simulink model "Fluid_Power_Control"  (R2024b)
settings: Solver=VariableStepAuto  StartTime=0.0  StopTime=10.0  RelTol=1e-3
model workspace (MAT data in the model file):
  b = 3
  m = 3
undefined symbols (not defined in the file): A, B, FL, kc, kq, ms, V
settings Model: Creator=audreyday  LastModifiedBy=audreyday

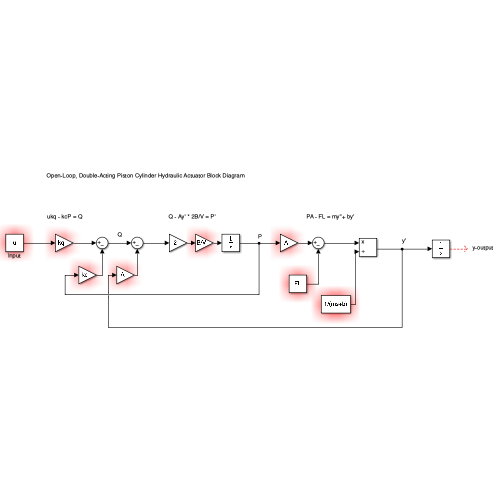
[thumbnail: Simulink's stored preview of the top-level diagram]
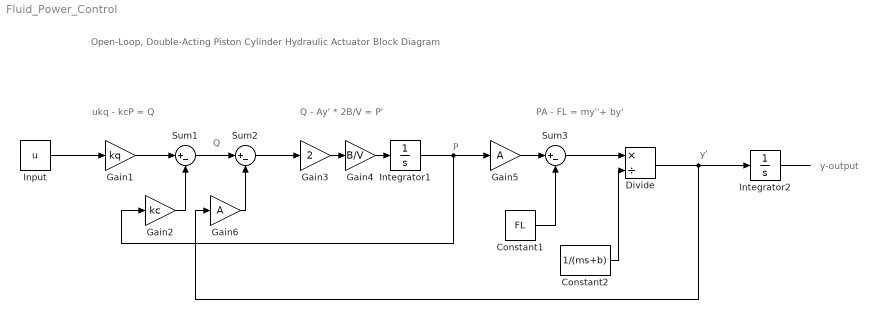
== system Fluid_Power_Control ==
  note: Open-Loop, Double-Acting Piston Cylinder Hydraulic Actuator Block Diagram
  note: y'
  note: PA - FL = my''+ by'
  note: P
  note: Q - Ay' * 2B/V = P'
  note: y-output
  note: ukq - kcP = Q
  note: Q
  Constant1 : Constant  Value=FL
  Constant2 : Constant  Value=1/(ms+b)
  Divide : Product  Inputs=*/
  Gain1 : Gain  Gain=kq
  Gain2 : Gain  Gain=kc
  Gain3 : Gain  Gain=2
  Gain4 : Gain  Gain=B/V
  Gain5 : Gain  Gain=A
  Gain6 : Gain  Gain=A
  Input : Constant  Value=u
  Integrator1 : Integrator
  Integrator2 : Integrator
  Sum1 : Sum  Inputs=|+-
  Sum2 : Sum  Inputs=|+-
  Sum3 : Sum  Inputs=|+-
  wires:
  Input/1 -> Gain1/1
  Gain1/1 -> Sum1/1
  Sum1/1 -> Sum2/1
  Gain2/1 -> Sum1/2
  Gain3/1 -> Gain4/1
  Sum2/1 -> Gain3/1
  Gain4/1 -> Integrator1/1
  Integrator1/1 -> Gain5/1, Gain2/1
  Gain5/1 -> Sum3/1
  Constant1/1 -> Sum3/2
  Gain6/1 -> Sum2/2
  Sum3/1 -> Divide/1
  Constant2/1 -> Divide/2
  Divide/1 -> Gain6/1, Integrator2/1
  Integrator2/1 -> ?
